simulink model "auto_pilot_udp"  (R2022b)
settings: Solver=FixedStepAuto  StartTime=0.0  StopTime=Inf  FixedStep=0.001  RelTol=1e-3  EnableMultiTasking=on
InitFcn:
  | clear mex
model workspace (MAT data in the model file):
  worldsim_instance : object (value not decoded)
values from neighbouring files (symbols this model uses):
  ACC_Adaptive_D = 0    [AutoPilot_parameters.m]    (also in ap_ini_param.mat; ap_initialModel.sldd = 0.0)
  ACC_Adaptive_I = 0    [AutoPilot_parameters.m]    (also in ap_ini_param.mat; ap_initialModel.sldd = 0.0)
  ACC_Adaptive_P = [5 7.5]    [AutoPilot_parameters.m]    (also in ap_ini_param.mat; ap_initialModel.sldd = 5.0 7.5)
  ACC_Classic_I = 5    [AutoPilot_parameters.m]    (also in ap_ini_param.mat; ap_initialModel.sldd = 5.0)
  ACC_Classic_P = 15    [AutoPilot_parameters.m]    (also in ap_ini_param.mat; ap_initialModel.sldd = 15.0)
  ACC_MaxBrake = 50    [AutoPilot_parameters.m]    (also in ap_ini_param.mat; ap_initialModel.sldd = 50.0)
  ACC_MaxThrottle = 130    [AutoPilot_parameters.m]    (also in ap_ini_param.mat = 80; ap_initialModel.sldd = 130.0)
  ACC_Module_Activity_Flag = 1    [AutoPilot_parameters.m]    (also in ap_ini_param.mat; ap_initialModel.sldd = 1.0)
  ACC_Ready_Speed = 30    [AutoPilot_parameters.m]    (also in ap_ini_param.mat; ap_initialModel.sldd = 30.0)
  ACC_SensorMaxDistance = 250    [AutoPilot_parameters.m]    (also in ap_ini_param.mat = 120; ap_initialModel.sldd = 250.0)
  ACC_Speed_Distance_control = 3    [AutoPilot_parameters.m]    (also in ap_ini_param.mat; ap_initialModel.sldd = 3.0)
  ACC_Speed_Distance_Gain = [0.1 0.15 0.2 0.25]    [AutoPilot_parameters.m]    (also in ap_ini_param.mat; ap_initialModel.sldd = 0.1 0.15 0.2 0.25)
  ADAS_Control_Mode = 1    [AutoPilot_parameters.m]    (also in ap_ini_param.mat; ap_initialModel.sldd = 1.0)
  AEB_Alarm_Freq = 5    [AutoPilot_parameters.m]    (also in ap_ini_param.mat; ap_initialModel.sldd = 5.0)
  AEB_Distance_To_Collision_Brake = 5    [AutoPilot_parameters.m]    (also in ap_ini_param.mat; ap_initialModel.sldd = 5.0)
  AEB_Freq_Hz = Sensor_Freq_worldsim/2    (= 25)    [AutoPilot_parameters.m]    (also in ap_ini_param.mat; ap_initialModel.sldd = 25.0)
  AEB_Gain = [1 1]    [AutoPilot_parameters.m]    (also in ap_ini_param.mat; ap_initialModel.sldd = 1.0 1.0)
  AEB_Gain_set = 60    [AutoPilot_parameters.m]    (also in ap_ini_param.mat; ap_initialModel.sldd = 60.0)
  AEB_Gain_set_mult = 0.03    [AutoPilot_parameters.m]    (also in ap_ini_param.mat; ap_initialModel.sldd)
  AEB_Max_Decel = [8 15]    [AutoPilot_parameters.m]    (also in ap_ini_param.mat; ap_initialModel.sldd = 8.0 15.0)
  AEB_Max_Speed = 150    [AutoPilot_parameters.m]    (also in ap_ini_param.mat = 100; ap_initialModel.sldd = 150.0)
  AEB_Min_Distance_at_Stop = 1    [AutoPilot_parameters.m]    (also in ap_ini_param.mat; ap_initialModel.sldd = 1.0)
  AEB_Module_Activity_Flag = 1    [AutoPilot_parameters.m]    (also in ap_ini_param.mat; ap_initialModel.sldd = 1.0)
  AEB_Pedestrian_type = 68    [AutoPilot_parameters.m]    (also in ap_ini_param.mat; ap_initialModel.sldd = 68.0)
  AEB_Steer_Max = 180    [AutoPilot_parameters.m]    (also in ap_ini_param.mat; ap_initialModel.sldd = 180.0)
  AP_Activity_Flag = 1    [AutoPilot_parameters.m]    (also in ap_ini_param.mat; ap_initialModel.sldd = 1.0)
  AP_D = [0.3 0.3]    [AutoPilot_parameters.m]    (also in ap_ini_param.mat; ap_initialModel.sldd = 0.3 0.3)
  AP_Dyn_Rate_Limiter_Gain = 0.1    [AutoPilot_parameters.m]    (also in ap_ini_param.mat; ap_initialModel.sldd)
  AP_Dyn_Rate_Limiter_Power = 10    [AutoPilot_parameters.m]    (also in ap_ini_param.mat; ap_initialModel.sldd = 10.0)
  AP_Error_Max = 3    [AutoPilot_parameters.m]    (also in ap_ini_param.mat; ap_initialModel.sldd = 3.0)
  AP_Freq_Hz = Sensor_Freq_worldsim    (= 50)    [AutoPilot_parameters.m]    (also in ap_ini_param.mat; ap_initialModel.sldd = 50.0)
  AP_I = [0.05 0.05]    [AutoPilot_parameters.m]    (also in ap_ini_param.mat; ap_initialModel.sldd = 0.05 0.05)
  AP_Max_Error_dydt_Disable = 0.5    [AutoPilot_parameters.m]    (also in ap_ini_param.mat; ap_initialModel.sldd)
  AP_On_Request_Time = 0.01    [AutoPilot_parameters.m]    (also in ap_ini_param.mat; ap_initialModel.sldd)
  AP_P = [0.2 0.2]    [AutoPilot_parameters.m]    (also in ap_ini_param.mat; ap_initialModel.sldd = 0.2 0.2)
  AP_Steer_Error_Max = 0.7    [AutoPilot_parameters.m]    (also in ap_ini_param.mat; ap_initialModel.sldd)
  AP_Steer_Rate_Max_radps = 1    [AutoPilot_parameters.m]    (also in ap_ini_param.mat; ap_initialModel.sldd = 1.0)
  AP_Transition_Rate = 0.5    [AutoPilot_parameters.m]    (also in ap_ini_param.mat; ap_initialModel.sldd)
  butter_a = [1 -1.9911142922 0.991153595869]    [ap_ini_param.mat]    (also in ap_initialModel.sldd = 1.0 -1.9911142922016536 0.99115359586893548)
  butter_a_lka_out = 1.0 -1.5610180758007179 0.641351538057563    [ap_initialModel.sldd]
  butter_b = [9.82591682048e-06 1.9651833641e-05 9.82591682048e-06]    [ap_ini_param.mat]    (also in ap_initialModel.sldd = 9.825916820482009E-6 1.9651833640964018E-5 9.825916820482009)
  butter_b_lka_out = 0.020083365564211246 0.040166731128422492 0.020083365564211246    [ap_initialModel.sldd]
  Lane_Width = 3.7    [AutoPilot_parameters.m]    (also in ap_ini_param.mat; ap_initialModel.sldd)
  LDW_Activity_Flag = 1    [ap_ini_param.mat]    (also in ap_initialModel.sldd = 1.0)
  LDW_Freq_Hz = 50    [ap_ini_param.mat]    (also in ap_initialModel.sldd = 50.0)
  LDW_LaneGap_dydt_Warning = 50    [ap_ini_param.mat]    (also in ap_initialModel.sldd = 50.0)
  LDW_LaneGap_Warning = [0.5 0.25]    [ap_ini_param.mat]    (also in ap_initialModel.sldd = 0.5 0.25)
  LDW_Min_Speed = 60    [ap_ini_param.mat]    (also in ap_initialModel.sldd = 60.0)
  LDW_Steer_Vibration_Amplitude = 5    [ap_ini_param.mat]    (also in ap_initialModel.sldd = 5.0)
  LDW_Steer_Vibration_Freq = 25    [ap_ini_param.mat]    (also in ap_initialModel.sldd = 25.0)
  LKA_Activity_Flag = 1    [ap_ini_param.mat]    (also in ap_initialModel.sldd = 1.0)
  LKA_D = [0.2 0.3]    [ap_ini_param.mat]    (also in ap_initialModel.sldd = 0.2 0.3)
  LKA_Dyn_Rate_Limiter_Gain = 0.1    [ap_ini_param.mat]    (also in ap_initialModel.sldd)
  LKA_Dyn_Rate_Limiter_Power = 10    [ap_ini_param.mat]    (also in ap_initialModel.sldd = 10.0)
  LKA_Error_dydt_Off = 1    [ap_ini_param.mat]    (also in ap_initialModel.sldd = 1.0)
  LKA_Error_Max = 3    [ap_ini_param.mat]    (also in ap_initialModel.sldd = 3.0)
  LKA_Error_Off = 0.5    [ap_ini_param.mat]    (also in ap_initialModel.sldd)
  LKA_Freq_Hz = 50    [ap_ini_param.mat]    (also in ap_initialModel.sldd = 50.0)
  LKA_I = [0.025 0.05]    [ap_ini_param.mat]    (also in ap_initialModel.sldd = 0.025 0.05)
  LKA_Lane_Gap_Activate = [0.25 0.125]    [ap_ini_param.mat]    (also in ap_initialModel.sldd = 0.25 0.125)
  LKA_Lane_Gap_dydt_Activate = 50    [ap_ini_param.mat]    (also in ap_initialModel.sldd = 50.0)
  LKA_Min_Speed = 60    [ap_ini_param.mat]    (also in ap_initialModel.sldd = 60.0)
  LKA_On_Display_Freq = 5    [ap_ini_param.mat]    (also in ap_initialModel.sldd = 5.0)
  LKA_P = [0.1 0.2]    [ap_ini_param.mat]    (also in ap_initialModel.sldd = 0.1 0.2)
  LKA_Steer_Rate_Max_radps = 1    [ap_ini_param.mat]    (also in ap_initialModel.sldd = 1.0)
  No_Target_Display_Value = 0    [AutoPilot_parameters.m]    (also in ap_ini_param.mat; ap_initialModel.sldd = 0.0)
  radar_source = 2    [AutoPilot_parameters.m]    (also in ap_ini_param.mat; ap_initialModel.sldd = 2.0)
  Sensor_Freq_worldsim = 50    [AutoPilot_parameters.m]    (also in ap_ini_param.mat; ap_initialModel.sldd = 50.0; launcher.m)
  stop_number_collisions = 10.0    [ap_initialModel.sldd]    (also in launcher.m = 10)
  stop_speed = 0.001    [ap_initialModel.sldd]    (also in launcher.m)
  stop_time = 12.0    [ap_initialModel.sldd]    (also in launcher.m = 12)
  vehicle_width = 2.2    [AutoPilot_parameters.m]    (also in ap_ini_param.mat = 1.86; ap_initialModel.sldd)
undefined symbols (not defined in the file or in its folder): blockPlatform, HOST, light_brake_center, light_brake_left, light_brake_right
libraries: simulink x103, simwbSfunlib x35, slpidlib x5, viworldsim_lib x5
(part 4 of 5)

== system auto_pilot_udp/AP/AP_Logic/Discrete PID Controller2 ==
  In1 : Inport
  In2 : Inport  Port=2
  In4 : Inport  Port=3
  ADAS_Control_Mode : Constant  Value=ADAS_Control_Mode
  AP_D(1)(1) : Constant  Value=AP_D(1)
  AP_D(2)(1)1 : Constant  Value=AP_D(2)
  AP_I(1)(1) : Constant  Value=AP_I(1)
  AP_I(2)(1)1 : Constant  Value=AP_I(2)
  AP_P(1)(1) : Constant  Value=AP_P(1)
  AP_P(2)(1)1 : Constant  Value=AP_P(2)
  Constant : Constant  Value=0
  Demux : Demux  Outputs=3
  Discrete PID Controller2 : slpidlib/PID Controller  Controller=PID  Form=Parallel  TimeDomain=Discrete-time  UseExternalTs=off  SampleTime=1/AP_Freq_Hz  IntegratorMethod=Forward Euler  FilterMethod=Forward Euler  ControllerParametersSource=external  P=AP_P  I=AP_I  UseKiTs=off  D=AP_D  N=100  UseFilter=off  TunerSelectOption=Transfer Function Based (PID Tuner App)  InitialConditionSource=external  InitialConditionForIntegrator=0  InitialConditionForFilter=0  DifferentiatorICPrevScaledInput=0  ExternalReset=either  TrackingMode=off  Kt=1  LimitOutput=off  SatLimitsSource=internal  UpperSaturationLimit=ACC_MaxThrottle  LowerSaturationLimit=-ACC_MaxBrake  LinearizeAsGain=off  AntiWindupMode=back-calculation  Kb=1  LimitIntegrator=off  UpperIntegratorSaturationLimit=inf  LowerIntegratorSaturationLimit=-inf  POutMin=[]  POutMax=[]  IOutMin=[]  IOutMax=[]  DOutMin=[]  DOutMax=[]  NOutMin=[]  NOutMax=[]  SumOutMin=[]  SumOutMax=[]  SaturationOutMin=[]  SaturationOutMax=[]  PParamMin=[]  PParamMax=[]  IParamMin=[]  IParamMax=[]  DParamMin=[]  DParamMax=[]  NParamMin=[]  NParamMax=[]  KbParamMin=[]  KbParamMax=[]  KtParamMin=[]  KtParamMax=[]  KbOutMin=[]  KbOutMax=[]  KtOutMin=[]  KtOutMax=[]  IntegratorOutMin=[]  IntegratorOutMax=[]  FilterOutMin=[]  FilterOutMax=[]  SumI1OutMin=[]  SumI1OutMax=[]  SumI2OutMin=[]  SumI2OutMax=[]  SumI3OutMin=[]  SumI3OutMax=[]  SumI4OutMin=[]  SumI4OutMax=[]  SumDOutMin=[]  SumDOutMax=[]  DifferentiatorOutMin=[]  DifferentiatorOutMax=[]  FilterDiffOutCoefMin=[]  FilterDiffOutCoefMax=[]  ReciprocalOutMin=[]  ReciprocalOutMax=[]  SumDenOutMin=[]  SumDenOutMax=[]  SumNumOutMin=[]  SumNumOutMax=[]  DivideOutMin=[]  DivideOutMax=[]  UdiffTsProdOutMin=[]  UdiffTsProdOutMax=[]  NTsProdOutMin=[]  NTsProdOutMax=[]  UintegralTsProdOutMin=[]  UintegralTsProdOutMax=[]  UngainTsProdOutMin=[]  UngainTsProdOutMax=[]  ClampingZeroOutDataTypeStr=Inherit: Inherit via back propagation  ClampingZeroOutMin=[]  ClampingZeroOutMax=[]  FilterDenConstantOutDataTypeStr=Inherit: Inherit via back propagation  FilterDenConstantOutMin=[]  FilterDenConstantOutMax=[]  PCopyOutDataTypeStr=Inherit: Inherit via back propagation  PCopyOutMin=[]  PCopyOutMax=[]  NCopyOutDataTypeStr=Inherit: Inherit via back propagation  NCopyOutMin=[]  NCopyOutMax=[]  IntegratorContinuousStateAttributes=''  IntegratorStateMustResolveToSignalObject=off  IntegratorRTWStateStorageClass=Auto  FilterContinuousStateAttributes=''  FilterStateMustResolveToSignalObject=off  FilterRTWStateStorageClass=Auto  ParallelPVariant=ExternalParameters  IdealPVariant=Disabled  IVariant=ExternalParameters  DVariant=ExternalParameters  IntegratorVariant=Discrete  SatVariant=Disabled  AWVariant=Passthrough  PCopyVariant=Disabled  TRVariant=Disabled  FdbkBlocksVariant=Forward  IdealPFdbkVariant=Disabled  SatFdbkVariant=Disabled  DerivativeFilterVariant=Differentiator  NVariant=Passthrough  NCopyVariant=Disabled_SignalSpec  FilterICVariant=ExternalICs  IntegratorICVariant=ExternalICs  ExternalResetVariant=ExternalReset  TRSumVariant=Passthrough  SumFdbkVariant=Disabled  SumVariant=Sum_PID  TsampFilterVariant=InternalTs  TsampNgainVariant=Passthrough  TsampIntegralVariant=Passthrough  ExternalSaturationOutDataTypeStr=Inherit: Same as second input
  Multiport Switch : MultiPortSwitch  Inputs=2  DataPortForDefault=Additional data port  DiagnosticForDefault=None  SaturateOnIntegerOverflow=off  InputSameDT=off
  Mux : Mux  Inputs=3
  Mux1 : Mux  Inputs=3
  Out1 : Outport  VectorParamsAs1DForOutWhenUnconnected=off
  wires:
  Constant/1 -> Discrete PID Controller2/7
  In2/1 -> Discrete PID Controller2/5
  Discrete PID Controller2/1 -> Out1/1
  In4/1 -> Discrete PID Controller2/6
  In1/1 -> Discrete PID Controller2/1
  AP_P(1)(1)/1 -> Mux/1
  ADAS_Control_Mode/1 -> Multiport Switch/1
  Mux1/1 -> Multiport Switch/3
  Mux/1 -> Multiport Switch/4, Multiport Switch/2
  AP_I(1)(1)/1 -> Mux/2
  AP_D(1)(1)/1 -> Mux/3
  AP_P(2)(1)1/1 -> Mux1/1
  AP_I(2)(1)1/1 -> Mux1/2
  AP_D(2)(1)1/1 -> Mux1/3
  Multiport Switch/1 -> Demux/1
  Demux/2 -> Discrete PID Controller2/3
  Demux/1 -> Discrete PID Controller2/2
  Demux/3 -> Discrete PID Controller2/4

== system auto_pilot_udp/AP/AP_Logic/Subsystem ==
  Clock : Inport
  Input_Signal : Inport  Port=2
  Delay : Delay  DelayLength=1000/AP_Freq_Hz  InitialCondition=-1/AP_Freq_Hz
  Delay1 : Delay  DelayLength=1000/AP_Freq_Hz
  Delay2 : Delay  DelayLength=1000/AP_Freq_Hz
  Lookup Table Dynamic : simulink/Lookup Tables/Lookup Table Dynamic  LookUpMeth=Interpolation-Use End Values  OutDataType=fixdt('double')  OutScaling=[]  OutputDataTypeScalingMode=Specify via dialog  OutDataTypeStr=fixdt('double')  DoSatur=off
  Vector Concatenate : Concatenate
  Vector Concatenate1 : Concatenate
  Zero-Order Hold1 : ZeroOrderHold  SampleTime=1/AP_Freq_Hz
  Zero-Order Hold2 : ZeroOrderHold  SampleTime=1/AP_Freq_Hz
  Zero-Order Hold3 : ZeroOrderHold  SampleTime=1e-3
  Zero-Order Hold4 : ZeroOrderHold  SampleTime=1e-3
  1kHz_Interpolation : Outport  VectorParamsAs1DForOutWhenUnconnected=off
  wires:
  Input_Signal/1 -> Zero-Order Hold1/1
  Zero-Order Hold1/1 -> Zero-Order Hold4/1
  Zero-Order Hold3/1 -> Delay/1, Vector Concatenate/2
  Zero-Order Hold2/1 -> Zero-Order Hold3/1
  Delay/1 -> Vector Concatenate/1
  Delay1/1 -> Lookup Table Dynamic/1
  Delay2/1 -> Vector Concatenate1/1
  Zero-Order Hold4/1 -> Delay2/1, Vector Concatenate1/2
  Vector Concatenate1/1 -> Lookup Table Dynamic/3
  Vector Concatenate/1 -> Lookup Table Dynamic/2
  Clock/1 -> Delay1/1, Zero-Order Hold2/1
  Lookup Table Dynamic/1 -> 1kHz_Interpolation/1

== system auto_pilot_udp/INPUT/Inputs for CRT/Clutch_manager ==
  throttle : Inport
  Cast To Double : DataTypeConversion  OutDataTypeStr=double  SaturateOnIntegerOverflow=off  RndMeth=Floor
  Compare To Constant4 : simulink/Logic and Bit Operations/Compare To Constant  relop===  const=0  OutDataTypeStr=boolean
  clutch : Outport
  wires:
  Compare To Constant4/1 -> Cast To Double/1
  Cast To Double/1 -> clutch/1  "clutch"
  throttle/1 -> Compare To Constant4/1

== system auto_pilot_udp/OUTPUT/WorldSim_Sensor_Outputs/Radar_selection ==
  note: assignement
  Bus Creator : BusCreator  Inputs=12
  Constant1 : Constant  Value=radar_source
  Demux : Demux  Outputs=3
  Demux1 : Demux
  Demux2 : Demux
  Demux3 : Demux
  Multiport Switch : MultiPortSwitch  Inputs=2  SaturateOnIntegerOverflow=off  InputSameDT=off
  Terminator : Terminator
  tag scope: SensorTargets_300000_azimuthInSensor_mux=global, SensorTargets_300000_distanceToCollision_mux=global, SensorTargets_300000_id_mux=global, SensorTargets_300000_type_mux=global, SensorTargets_300001_azimuthInSensor_mux=global, SensorTargets_300001_distanceToCollision_mux=global, SensorTargets_300001_id_mux=global, SensorTargets_300001_type_mux=global, SensorTargets_300002_azimuthInSensor_mux=global, SensorTargets_300002_distanceToCollision_mux=global, SensorTargets_300002_id_mux=global, SensorTargets_300002_type_mux=global
  wires:
  [radar_virtual] -> Multiport Switch/3
  [radar_multiagent] -> Multiport Switch/2
  Constant1/1 -> Multiport Switch/1
  Multiport Switch/1 -> Demux/1
  Demux1/1 -> [SensorTargets_300000_id_mux]
  Demux3/4 -> [SensorTargets_300002_type_mux]
  Demux3/1 -> [SensorTargets_300002_id_mux]
  Demux1/4 -> [SensorTargets_300000_type_mux]
  Demux3/2 -> [SensorTargets_300002_distanceToCollision_mux]
  Demux2/3 -> [SensorTargets_300001_azimuthInSensor_mux]
  Demux1/2 -> [SensorTargets_300000_distanceToCollision_mux]
  Demux/1 -> Demux1/1
  Demux1/3 -> [SensorTargets_300000_azimuthInSensor_mux]
  Demux2/2 -> [SensorTargets_300001_distanceToCollision_mux]
  Demux3/3 -> [SensorTargets_300002_azimuthInSensor_mux]
  Demux2/4 -> [SensorTargets_300001_type_mux]
  Demux/3 -> Demux3/1
  Demux/2 -> Demux2/1
  Demux2/1 -> [SensorTargets_300001_id_mux]
  [SensorTargets_300000_id_mux] -> Bus Creator/1
  [SensorTargets_300000_distanceToCollision_mux] -> Bus Creator/2
  [SensorTargets_300000_azimuthInSensor_mux] -> Bus Creator/3
  [SensorTargets_300000_type_mux] -> Bus Creator/4
  [SensorTargets_300001_id_mux] -> Bus Creator/5
  [SensorTargets_300001_distanceToCollision_mux] -> Bus Creator/6
  [SensorTargets_300001_azimuthInSensor_mux] -> Bus Creator/7
  [SensorTargets_300001_type_mux] -> Bus Creator/8
  [SensorTargets_300002_id_mux] -> Bus Creator/9
  [SensorTargets_300002_distanceToCollision_mux] -> Bus Creator/10
  [SensorTargets_300002_azimuthInSensor_mux] -> Bus Creator/11
  [SensorTargets_300002_type_mux] -> Bus Creator/12
  Bus Creator/1 -> Terminator/1

== system auto_pilot_udp/OUTPUT/WorldSim_Sensor_Outputs/Subsystem ==
  Multiagent_radar_matrix [dimension: 64x7] : Inport
  Virtual_camera_radar_matrix [dimension: 10x10] : Inport  Port=2
  BSD_virtual_camera_matrix [dimension: 10x10] : Inport  Port=3
  Left_lane_distance [dimension: 1x1] : Inport  Port=4
  Right_lane_distance [dimension: 1x1] : Inport  Port=5
  Lane_detector_message_count [dimension: 1x1] : Inport  Port=6
  Semitrack : Constant  Value=vehicle_width/2
  Terminator : Terminator
  Terminator1 : Terminator
  bsd setection from ostacle recognition : Subsystem
  lane marking acquisition : Subsystem
  "multiagent radar SimpleRadar_... are single double representing id, yaw, range, power_db, range_rate, yaw_rate, status" : Subsystem
  "obstacle detection " : Subsystem
  tag scope: frame_worldsim_left=global, frame_worldsim_right=global
  wires:
  Semitrack/1 -> lane marking acquisition/1(Semitrack), bsd setection from ostacle recognition/1(semitrack)
  Virtual_camera_radar_matrix [dimension: 10x10]/1 -> "obstacle detection "/1(Virtual_camera_obstacle_matrix)
  BSD_virtual_camera_matrix [dimension: 10x10]/1 -> bsd setection from ostacle recognition/2(BSD_matrix_obstalces)
  Left_lane_distance [dimension: 1x1]/1 -> lane marking acquisition/2(Left_lane_marking)
  Right_lane_distance [dimension: 1x1]/1 -> lane marking acquisition/3(Right_lane_marking)
  Multiagent_radar_matrix [dimension: 64x7]/1 -> "multiagent radar SimpleRadar_... are single double representing id, yaw, range, power_db, range_rate, yaw_rate, status"/1(Virtual_radar_obstacle_matrix)
  Lane_detector_message_count [dimension: 1x1]/1 -> [frame_worldsim_right], [frame_worldsim_left]
  [frame_worldsim_left] -> Terminator/1
  [frame_worldsim_right] -> Terminator1/1

== system auto_pilot_udp/VI-WorldSim Lights Manager/Lights/Default Lights Bus ==
  Bus Creator : BusCreator  Inputs=15
  Constant{,1..12,14..15} (15 alike) : Constant  Value=0
  Out1 : Outport  VectorParamsAs1DForOutWhenUnconnected=off
  wires:
  Bus Creator/1 -> Out1/1
  Constant12/1 -> Bus Creator/15  "light_daytime"
  Constant14/1 -> Bus Creator/13  "light_brake_center"
  Constant8/1 -> Bus Creator/9  "light_tail_left"
  Constant15/1 -> Bus Creator/14  "light_reverse"
  Constant2/1 -> Bus Creator/3  "light_high_beam_left"
  Constant5/1 -> Bus Creator/6  "light_indicator_right"
  Constant3/1 -> Bus Creator/4  "light_high_beam_right"
  Constant7/1 -> Bus Creator/8  "light_fog_right"
  Constant6/1 -> Bus Creator/7  "light_fog_left"
  Constant4/1 -> Bus Creator/5  "light_indicator_left"
  Constant1/1 -> Bus Creator/2  "light_low_beam_right"
  Constant/1 -> Bus Creator/1  "light_low_beam_left"
  Constant9/1 -> Bus Creator/10  "light_tail_right"
  Constant11/1 -> Bus Creator/12  "light_brake_right"
  Constant10/1 -> Bus Creator/11  "light_brake_left"

== system auto_pilot_udp/ACC/ACC_Logic/ACC_Speed_Controller/ACC_Speed_Distance_Gain ==
  note: this should be used when no varying distance is used
  In1 : Inport
  ACC_Speed_Distance_Gain : Gain  Gain=ACC_Speed_Distance_Gain(1)
  ACC_Speed_Distance_Gain1 : Gain  Gain=ACC_Speed_Distance_Gain(2)
  ACC_Speed_Distance_Gain2 : Gain  Gain=ACC_Speed_Distance_Gain(3)
  ACC_Speed_Distance_Gain3 : Gain  Gain=ACC_Speed_Distance_Gain(4)
  ADAS_Control_Mode : Constant  Value=ADAS_Control_Mode
  Cast To Double : DataTypeConversion  OutDataTypeStr=double  SaturateOnIntegerOverflow=off  RndMeth=Floor
  Detect Increase : simulink/Logic and Bit Operations/Detect Increase  vinit=0.0  OutDataTypeStr=boolean
  Detect Increase1 : simulink/Logic and Bit Operations/Detect Increase  vinit=0.0  OutDataTypeStr=boolean
  Gain : Gain  Gain=-1
  Memory : Memory  InitialCondition=ACC_Speed_Distance_control
  Multiport Switch : MultiPortSwitch  Inputs=4  DataPortForDefault=Additional data port  DiagnosticForDefault=None  SaturateOnIntegerOverflow=off  InputSameDT=off
  Saturation : Saturate  UpperLimit=4  LowerLimit=1
  Sum : Sum  Inputs=+++
  Terminator : Terminator
  Terminator1 : Terminator
  Out1 : Outport  VectorParamsAs1DForOutWhenUnconnected=off
  tag scope: ACC_distance_step=global
  wires:
  Multiport Switch/1 -> Out1/1
  In1/1 -> ACC_Speed_Distance_Gain3/1, ACC_Speed_Distance_Gain2/1, ACC_Speed_Distance_Gain1/1, ACC_Speed_Distance_Gain/1
  ACC_Speed_Distance_Gain/1 -> Multiport Switch/2
  ACC_Speed_Distance_Gain1/1 -> Multiport Switch/6, Multiport Switch/3
  ACC_Speed_Distance_Gain2/1 -> Multiport Switch/4
  ACC_Speed_Distance_Gain3/1 -> Multiport Switch/5
  [mode_minus] -> Detect Increase/1
  Detect Increase/1 -> Gain/1
  [mode_plus] -> Detect Increase1/1
  Sum/1 -> Multiport Switch/1, Memory/1, Cast To Double/1
  Memory/1 -> Saturation/1
  Saturation/1 -> Sum/3
  Detect Increase1/1 -> Sum/2
  Gain/1 -> Sum/1
  ADAS_Control_Mode/1 -> Terminator/1
  Cast To Double/1 -> [ACC_distance_step]
  [ACC_distance_step] -> Terminator1/1

== system auto_pilot_udp/ACC/ACC_Logic/ACC_Speed_Controller/tACC_PID ==
  In1 : Inport
  In2 : Inport  Port=2
  ACC_Adaptive_P : Constant  Value=ACC_Adaptive_P(1)
  ACC_Adaptive_P2 : Constant  Value=ACC_Adaptive_P(2)
  ADAS_Control_Mode : Constant  Value=ADAS_Control_Mode
  Constant : Constant  Value=0
  Multiport Switch : MultiPortSwitch  Inputs=2  DataPortForDefault=Additional data port  DiagnosticForDefault=None  SaturateOnIntegerOverflow=off  InputSameDT=off
  tACC_PID : slpidlib/PID Controller  Controller=PID  Form=Parallel  TimeDomain=Discrete-time  UseExternalTs=off  SampleTime=-1  IntegratorMethod=Forward Euler  FilterMethod=Forward Euler  ControllerParametersSource=external  P=ACC_Adaptive_P  I=ACC_Adaptive_I  UseKiTs=off  D=ACC_Adaptive_D  N=100  UseFilter=off  TunerSelectOption=Transfer Function Based (PID Tuner App)  InitialConditionSource=internal  InitialConditionForIntegrator=0  InitialConditionForFilter=0  DifferentiatorICPrevScaledInput=0  ExternalReset=either  TrackingMode=off  Kt=1  LimitOutput=on  SatLimitsSource=internal  UpperSaturationLimit=ACC_MaxThrottle  LowerSaturationLimit=-ACC_MaxBrake  LinearizeAsGain=off  AntiWindupMode=back-calculation  Kb=1  LimitIntegrator=off  UpperIntegratorSaturationLimit=inf  LowerIntegratorSaturationLimit=-inf  POutMin=[]  POutMax=[]  IOutMin=[]  IOutMax=[]  DOutMin=[]  DOutMax=[]  NOutMin=[]  NOutMax=[]  SumOutMin=[]  SumOutMax=[]  SaturationOutMin=[]  SaturationOutMax=[]  PParamMin=[]  PParamMax=[]  IParamMin=[]  IParamMax=[]  DParamMin=[]  DParamMax=[]  NParamMin=[]  NParamMax=[]  KbParamMin=[]  KbParamMax=[]  KtParamMin=[]  KtParamMax=[]  KbOutMin=[]  KbOutMax=[]  KtOutMin=[]  KtOutMax=[]  IntegratorOutMin=[]  IntegratorOutMax=[]  FilterOutMin=[]  FilterOutMax=[]  SumI1OutMin=[]  SumI1OutMax=[]  SumI2OutMin=[]  SumI2OutMax=[]  SumI3OutMin=[]  SumI3OutMax=[]  SumI4OutMin=[]  SumI4OutMax=[]  SumDOutMin=[]  SumDOutMax=[]  DifferentiatorOutMin=[]  DifferentiatorOutMax=[]  FilterDiffOutCoefMin=[]  FilterDiffOutCoefMax=[]  ReciprocalOutMin=[]  ReciprocalOutMax=[]  SumDenOutMin=[]  SumDenOutMax=[]  SumNumOutMin=[]  SumNumOutMax=[]  DivideOutMin=[]  DivideOutMax=[]  UdiffTsProdOutMin=[]  UdiffTsProdOutMax=[]  NTsProdOutMin=[]  NTsProdOutMax=[]  UintegralTsProdOutMin=[]  UintegralTsProdOutMax=[]  UngainTsProdOutMin=[]  UngainTsProdOutMax=[]  ClampingZeroOutDataTypeStr=Inherit: Inherit via back propagation  ClampingZeroOutMin=[]  ClampingZeroOutMax=[]  FilterDenConstantOutDataTypeStr=Inherit: Inherit via back propagation  FilterDenConstantOutMin=[]  FilterDenConstantOutMax=[]  PCopyOutDataTypeStr=Inherit: Inherit via back propagation  PCopyOutMin=[]  PCopyOutMax=[]  NCopyOutDataTypeStr=Inherit: Inherit via back propagation  NCopyOutMin=[]  NCopyOutMax=[]  IntegratorContinuousStateAttributes=''  IntegratorStateMustResolveToSignalObject=off  IntegratorRTWStateStorageClass=Auto  FilterContinuousStateAttributes=''  FilterStateMustResolveToSignalObject=off  FilterRTWStateStorageClass=Auto  ParallelPVariant=ExternalParameters  IdealPVariant=Disabled  IVariant=ExternalParameters  DVariant=ExternalParameters  IntegratorVariant=Discrete  SatVariant=Enabled  AWVariant=BackCalculation  PCopyVariant=Disabled  TRVariant=Disabled  FdbkBlocksVariant=Forward  IdealPFdbkVariant=Disabled  SatFdbkVariant=Disabled  DerivativeFilterVariant=Differentiator  NVariant=Passthrough  NCopyVariant=Disabled_SignalSpec  FilterICVariant=InternalICsDifferentiator  IntegratorICVariant=InternalICs  ExternalResetVariant=ExternalReset  TRSumVariant=Passthrough  SumFdbkVariant=Disabled  SumVariant=Sum_PID  TsampFilterVariant=InternalTs  TsampNgainVariant=Passthrough  TsampIntegralVariant=Passthrough  ExternalSaturationOutDataTypeStr=Inherit: Same as second input
  Out1 : Outport  VectorParamsAs1DForOutWhenUnconnected=off
  wires:
  tACC_PID/1 -> Out1/1
  In1/1 -> tACC_PID/1
  In2/1 -> tACC_PID/5
  ACC_Adaptive_P/1 -> Multiport Switch/4, Multiport Switch/2
  ADAS_Control_Mode/1 -> Multiport Switch/1
  ACC_Adaptive_P2/1 -> Multiport Switch/3
  Multiport Switch/1 -> tACC_PID/2
  Constant/1 -> tACC_PID/3, tACC_PID/4

== system auto_pilot_udp/ACC/ACC_Logic/ACC_Target_Acquisition/SensorTargets_300000_ClosestTargetDistance ==
  ACC_SensorMaxDistance : Constant  Value=ACC_SensorMaxDistance + 1
  Abs : Abs  SaturateOnIntegerOverflow=off
  MinMax : MinMax
  Switch : Switch  Criteria=u2 > Threshold  SaturateOnIntegerOverflow=off  InputSameDT=off
  Switch1 : Switch  Criteria=u2 > Threshold  Threshold=0.02  SaturateOnIntegerOverflow=off  InputSameDT=off
  tag scope: SensorTargets_300000_ClosestTargetDistance=global
  wires:
  [SensorTargets_300000_distanceToCollision_mux] -> Switch/1
  ACC_SensorMaxDistance/1 -> Switch/3
  MinMax/1 -> [SensorTargets_300000_ClosestTargetDistance]
  Switch1/1 -> Switch/2
  [SensorTargets_300000_InStraightLane_mux] -> Switch1/3
  [SensorTargets_300000_InCurvedLane_mux] -> Switch1/1
  [ACC_Input_Front_Axle_Steer] -> Abs/1
  Abs/1 -> Switch1/2
  Switch/1 -> MinMax/1

== system auto_pilot_udp/ACC/ACC_Logic/ACC_Target_Acquisition/SensorTargets_300000_ClosestTargetId ==
  note: if ws_radar is used or simple multiagent radar is used
  AND : Logic  AllPortsSameDT=off  OutDataTypeStr=boolean
  Compare To Constant : simulink/Logic and Bit Operations/Compare To Constant  relop=~=  const=1  OutDataTypeStr=boolean
  Compare To Constant1 : simulink/Logic and Bit Operations/Compare To Constant  relop=~=  const=1  OutDataTypeStr=boolean
  Compare To Constant2 : simulink/Logic and Bit Operations/Compare To Constant  relop===  const=121  OutDataTypeStr=boolean
  Compare To Constant3 : simulink/Logic and Bit Operations/Compare To Constant  relop===  const=3  OutDataTypeStr=boolean
  Constant : Constant  Value=0
  Constant1 : Constant  Value=radar_source
  Logical Operator : Logic  Operator=OR  Inputs=4  AllPortsSameDT=off  OutDataTypeStr=boolean
  Logical Operator1 : Logic  Operator=OR  AllPortsSameDT=off  OutDataTypeStr=boolean
  MinMax : MinMax  Function=max
  No_Target_Display_Value : Constant  Value=No_Target_Display_Value
  Product : Product
  Relational Operator : RelationalOperator  Operator===  OutDataTypeStr=boolean  InputSameDT=off
  Relational Operator1 : RelationalOperator  Operator=isNaN  OutDataTypeStr=boolean  InputSameDT=off
  Relational Operator2 : RelationalOperator  Operator=isInf  OutDataTypeStr=boolean  InputSameDT=off
  Switch : Switch  Criteria=u2 > Threshold  SaturateOnIntegerOverflow=off  InputSameDT=off
  Switch1 : Switch  Criteria=u2 > Threshold  SaturateOnIntegerOverflow=off  InputSameDT=off
  tag scope: ACC_Target_id=global
  wires:
  Product/1 -> MinMax/1
  Relational Operator/1 -> Product/2
  [SensorTargets_300000_id_mux] -> Product/1
  [SensorTargets_300000_ClosestTargetDistance] -> Relational Operator/2
  [SensorTargets_300000_distanceToCollision_mux] -> Relational Operator/1
  No_Target_Display_Value/1 -> Switch/1
  MinMax/1 -> Relational Operator2/1, Relational Operator1/1, Switch/3
  Switch/1 -> [ACC_Target_id]
  Logical Operator/1 -> Switch/2
  Relational Operator1/1 -> Logical Operator/3
  Relational Operator2/1 -> Logical Operator/2
  Compare To Constant/1 -> Logical Operator/4
  [ACC_Active] -> Logical Operator1/2
  [ACC_Ready] -> Logical Operator1/1
  Logical Operator1/1 -> Compare To Constant/1
  [SimpleRadar_status] -> Compare To Constant1/1
  Compare To Constant1/1 -> Switch1/3
  [SensorTargets_300000_ClosestTargetDistance] -> Compare To Constant2/1
  Compare To Constant2/1 -> AND/1
  Constant1/1 -> Compare To Constant3/1
  Compare To Constant3/1 -> AND/2, Switch1/2
  AND/1 -> Switch1/1
  Switch1/1 -> Logical Operator/1
  Constant/1 -> [SimpleRadar_status]

== system auto_pilot_udp/ACC/ACC_Logic/ACC_Target_Acquisition/SensorTargets_300000_InCurvedLane_mux ==
  Abs : Abs  SaturateOnIntegerOverflow=off
  Constant : Constant  Value=vehicle_width*0.8
  Gain : Gain
  Gain1 : Gain  Gain=1.3
  Lane_Width/2 : Constant  Value=Lane_Width/2
  Logical Operator : Logic  AllPortsSameDT=off  OutDataTypeStr=boolean
  MATLAB Function : MATLAB Function  TreatAsAtomicUnit=on
  MinMax : MinMax  Function=max
  Relational Operator : RelationalOperator  Operator=<  OutDataTypeStr=boolean  InputSameDT=off
  Relational Operator1 : RelationalOperator  Operator=>  OutDataTypeStr=boolean  InputSameDT=off
  Sum : Sum
  Sum1 : Sum  Inputs=-+
  Terminator : Terminator
  Terminator1 : Terminator
  Wrap To Zero : simulink/Discontinuities/Wrap To Zero  Threshold=10000
  Wrap To Zero1 : simulink/Discontinuities/Wrap To Zero  Threshold=10000
  tag scope: ACC_CurveRadius=global, ACC_CurveRadius_Target=global, SensorTargets_300000_InCurvedLane_mux=global
  wires:
  MATLAB Function/1(Radius) -> Abs/1
  MATLAB Function/2(Rn) -> Wrap To Zero1/1, Relational Operator/2, Relational Operator1/2
  Lane_Width/2/1 -> Gain1/1
  Sum1/1 -> Relational Operator/1
  Sum/1 -> Relational Operator1/1
  Relational Operator1/1 -> Logical Operator/1
  Relational Operator/1 -> Logical Operator/2
  Logical Operator/1 -> [SensorTargets_300000_InCurvedLane_mux]
  [Vehicle_wheelbase] -> MATLAB Function/2(wheelbase)
  [ACC_Input_Front_Axle_Steer] -> Gain/1
  [SensorTargets_300000_LateralDistance_mux] -> MATLAB Function/4(SensorTargets_300000_LateralDistance)
  [SensorTargets_300000_LongitudinalDistance_mux] -> MATLAB Function/3(SensorTargets_300000_LongitudinalDistance)
  Gain/1 -> MATLAB Function/1(Front_Axle_Steer)
  Wrap To Zero/1 -> [ACC_CurveRadius]
  Abs/1 -> Wrap To Zero/1, Sum/1, Sum1/2
  Wrap To Zero1/1 -> MinMax/1
  MinMax/1 -> [ACC_CurveRadius_Target]
  Gain1/1 -> Sum1/1, Sum/2
  Constant/1 -> [Vehicle_wheelbase]
  [ACC_CurveRadius_Target] -> Terminator/1
  [ACC_CurveRadius] -> Terminator1/1

== system auto_pilot_udp/ACC/ACC_Logic/ACC_Target_Acquisition/SensorTargets_300000_InStraightLane_mux ==
  Abs : Abs  SaturateOnIntegerOverflow=off
  Compare_to_Lane_Width_div2 : simulink/Logic and Bit Operations/Compare To Constant  relop=<=  const=Lane_Width/2  OutDataTypeStr=boolean
  tag scope: SensorTargets_300000_InStraightLane_mux=global
  wires:
  Compare_to_Lane_Width_div2/1 -> [SensorTargets_300000_InStraightLane_mux]
  Abs/1 -> Compare_to_Lane_Width_div2/1
  [SensorTargets_300000_LateralDistance_mux] -> Abs/1

== system auto_pilot_udp/ACC/ACC_Logic/ACC_Target_Acquisition/SensorTargets_300000_LateralDistance_mux ==
  Target_Lateral_Position : MATLAB Function  TreatAsAtomicUnit=on
  tag scope: SensorTargets_300000_LateralDistance_mux=global
  wires:
  Target_Lateral_Position/1(Target_Lateral_Position) -> [SensorTargets_300000_LateralDistance_mux]
  [SensorTargets_300000_distanceToCollision_mux] -> Target_Lateral_Position/1(Target_distance)
  [SensorTargets_300000_azimuthInSensor_mux] -> Target_Lateral_Position/2(Target_azimuth)

== system auto_pilot_udp/ACC/ACC_Logic/ACC_Target_Acquisition/SensorTargets_300000_LongitudinalDistance_mux ==
  Target_Longitudinal_Position : MATLAB Function  TreatAsAtomicUnit=on
  tag scope: SensorTargets_300000_LongitudinalDistance_mux=global
  wires:
  [SensorTargets_300000_distanceToCollision_mux] -> Target_Longitudinal_Position/1(Target_distance)
  [SensorTargets_300000_azimuthInSensor_mux] -> Target_Longitudinal_Position/2(Target_azimuth)
  Target_Longitudinal_Position/1(Target_Longitudinal_Position) -> [SensorTargets_300000_LongitudinalDistance_mux]

== system auto_pilot_udp/AEB/AEB_Logic/Target_XY_TimeToCollision/Target_Collision_Identifier_mux    ==
  Target_Y_Left_TimeToCollision : Inport
  Target_Y_Right_TimeToCollision : Inport  Port=2
  Target_X_TimeToCollision : Inport  Port=3
  Constant : Constant  Value=AEB_Gain_set
  Constant1 : Constant
  Gain : Gain  Gain=AEB_Gain(1)
  Gain1 : Gain  Gain=AEB_Gain(2)
  Gain2 : Gain  Gain=AEB_Gain_set_mult
  Logical Operator : Logic  AllPortsSameDT=off  OutDataTypeStr=boolean
  MinMax : MinMax  Inputs=2
  MinMax1 : MinMax  Function=max  Inputs=2
  Product : Product
  Product1 : Product
  Rate Transition : RateTransition  OutPortSampleTime=1/AEB_Freq_Hz
  Rate Transition1 : RateTransition  OutPortSampleTime=1/AEB_Freq_Hz
  Relational Operator : RelationalOperator  Operator=>  OutDataTypeStr=boolean  InputSameDT=off
  Relational Operator1 : RelationalOperator  Operator=<  OutDataTypeStr=boolean  InputSameDT=off
  Saturation : Saturate  UpperLimit=1.7  LowerLimit=0.8
  Sum : Sum  Inputs=+-
  Sum1 : Sum
  Target_Collision_Identifier : Outport  VectorParamsAs1DForOutWhenUnconnected=off
  wires:
  Relational Operator1/1 -> Logical Operator/1
  Relational Operator/1 -> Logical Operator/2
  MinMax/1 -> Gain/1
  Target_Y_Right_TimeToCollision/1 -> MinMax/2, MinMax1/2
  Target_X_TimeToCollision/1 -> Relational Operator1/2, Relational Operator/2
  Target_Y_Left_TimeToCollision/1 -> MinMax/1, MinMax1/1
  MinMax1/1 -> Gain1/1
  Constant/1 -> Sum/1
  [Vehicle_Speed] -> Rate Transition/1
  Gain/1 -> Product/2
  Gain1/1 -> Product1/2
  Constant1/1 -> Sum1/1
  Sum/1 -> Gain2/1
  Gain2/1 -> Sum1/2
  Sum1/1 -> Saturation/1
  Rate Transition/1 -> Sum/2
  Logical Operator/1 -> Rate Transition1/1
  Rate Transition1/1 -> Target_Collision_Identifier/1
  Product/1 -> Relational Operator1/1
  Saturation/1 -> Product1/1, Product/1
  Product1/1 -> Relational Operator/1

== system auto_pilot_udp/AEB/AEB_Logic/Target_XY_TimeToCollision/Target_X_TimeToCollision_mux ==
  Target_X_Distance : Inport
  Discrete Derivative : simulink/Discrete/Discrete Derivative  gainval=1.0  ICPrevScaledInput=0.0  OutMin=[]  OutMax=[]  OutDataType=fixdt(1, 16)  OutScaling=2^-10  DoSatur=off
  Div : Product  Inputs=*/
  Gain : Gain  Gain=-1
  MinMax : MinMax
  Saturation : Saturate  UpperLimit=-1e-6  LowerLimit=-inf
  Terminator : Terminator
  Target_X_TimeToCollision : Outport  VectorParamsAs1DForOutWhenUnconnected=off
  tag scope: AEB_Min_Target_X_Speed=global
  wires:
  Target_X_Distance/1 -> Div/1, Discrete Derivative/1
  Div/1 -> Gain/1
  Gain/1 -> Target_X_TimeToCollision/1
  Discrete Derivative/1 -> Saturation/1
  MinMax/1 -> [AEB_Min_Target_X_Speed]
  Saturation/1 -> MinMax/1, Div/2
  [AEB_Min_Target_X_Speed] -> Terminator/1

== system auto_pilot_udp/AEB/AEB_Logic/Target_XY_TimeToCollision/Target_Y_TimeToCollision_mux ==
  Target_Y_Distance : Inport
  Discrete Derivative1 : simulink/Discrete/Discrete Derivative  gainval=1.0  ICPrevScaledInput=0.0  OutMin=[]  OutMax=[]  OutDataType=fixdt(1, 16)  OutScaling=2^-10  DoSatur=off
  Discrete Derivative2 : simulink/Discrete/Discrete Derivative  gainval=1.0  ICPrevScaledInput=0.0  OutMin=[]  OutMax=[]  OutDataType=fixdt(1, 16)  OutScaling=2^-10  DoSatur=off
  Discrete Derivative3 : simulink/Discrete/Discrete Derivative  gainval=1.0  ICPrevScaledInput=0.0  OutMin=[]  OutMax=[]  OutDataType=fixdt(1, 16)  OutScaling=2^-10  DoSatur=off
  Div1 : Product  Inputs=*/  OutMin=[1e-6]
  Div2 : Product  Inputs=*/
  Gain1 : Gain  Gain=-1
  Gain2 : Gain  Gain=-1
  Lane_Left_Edge_Y_Distance : Constant  Value=1.5
  Lane_Right_Edge_Y_Distance : Constant  Value=-1.5
  MinMax : MinMax
  Saturation : Saturate  UpperLimit=-1e-6  LowerLimit=-inf
  Saturation1 : Saturate  UpperLimit=-1e-6  LowerLimit=-inf
  Sum : Sum  Inputs=+-
  Sum1 : Sum  Inputs=-+
  Terminator : Terminator
  Target_Y_Left_TimeToCollision : Outport  VectorParamsAs1DForOutWhenUnconnected=off
  Target_Y_Right_TimeToCollision : Outport  Port=2  VectorParamsAs1DForOutWhenUnconnected=off
  tag scope: AEB_Min_Target_Y_Speed=global
  wires:
  Discrete Derivative2/1 -> Saturation/1
  Lane_Left_Edge_Y_Distance/1 -> Sum/2
  Target_Y_Distance/1 -> Discrete Derivative3/1, Sum/1, Sum1/2
  Div1/1 -> Gain1/1
  Sum/1 -> Discrete Derivative1/1, Div1/1
  Sum1/1 -> Discrete Derivative2/1, Div2/1
  Discrete Derivative1/1 -> Saturation1/1
  Div2/1 -> Gain2/1
  Gain2/1 -> Target_Y_Left_TimeToCollision/1
  Gain1/1 -> Target_Y_Right_TimeToCollision/1
  Lane_Right_Edge_Y_Distance/1 -> Sum1/1
  Discrete Derivative3/1 -> MinMax/1
  MinMax/1 -> [AEB_Min_Target_Y_Speed]
  Saturation/1 -> Div2/2
  Saturation1/1 -> Div1/2
  [AEB_Min_Target_Y_Speed] -> Terminator/1

== system auto_pilot_udp/OUTPUT/WorldSim_Sensor_Outputs/Subsystem/bsd setection from ostacle recognition ==
  semitrack : Inport
  BSD_matrix_obstalces : Inport  Port=2
  Compare To Constant : simulink/Logic and Bit Operations/Compare To Constant  relop=>  const=30  OutDataTypeStr=boolean
  MATLAB Function3 : MATLAB Function  TreatAsAtomicUnit=on
  Product : Product
  Product1 : Product
  Terminator : Terminator
  Terminator1 : Terminator
  tag scope: BSD_left_ws=global, BSD_right_ws=global
  wires:
  Compare To Constant/1 -> Product1/1, Product/1
  BSD_matrix_obstalces/1 -> MATLAB Function3/1(u)
  Product/1 -> [BSD_left_ws]
  Product1/1 -> [BSD_right_ws]
  MATLAB Function3/2(right) -> Product1/2
  [Vehicle_Speed] -> Compare To Constant/1
  MATLAB Function3/1(left) -> Product/2
  semitrack/1 -> MATLAB Function3/2(semitrack)
  [BSD_left_ws] -> Terminator/1
  [BSD_right_ws] -> Terminator1/1

== system auto_pilot_udp/OUTPUT/WorldSim_Sensor_Outputs/Subsystem/lane marking acquisition ==
  note: . data from ws sensor are y data. sign is negative for right lane, positive for left lane. status = 1 means data are ok. vehicle track is used to make this data as similar as possible to scaner data
  Semitrack : Inport
  Left_lane_marking : Inport  Port=2
  Right_lane_marking : Inport  Port=3
  Bus Creator : BusCreator  Inputs=2
  Constant : Constant  Value=0
  Discrete Filter : DiscreteFilter  Numerator=[butter_b]  Denominator=[butter_a]  SampleTime=1e-3
  Discrete Filter1 : DiscreteFilter  Numerator=[butter_b]  Denominator=[butter_a]  SampleTime=1e-3
  Gain2 : Gain  Gain=-1
  Pulse Generator : DiscretePulseGenerator  PulseType=Time based  Period=1/Sensor_Freq_worldsim  PulseWidth=Sensor_Freq_worldsim*100/1000
  Sum : Sum  Inputs=-+
  Sum1 : Sum  Inputs=-+
  Terminator : Terminator
  Terminator1 : Terminator
  Terminator2 : Terminator
  derivation_speed : Subsystem
  filtering : DiscreteFilter  Numerator=[butter_b]  Denominator=[butter_a]  SampleTime=1e-3
  tag scope: LaneGap_left_ws=global, LaneGap_right_ws=global, LaneGap_speed_left_ws=global, LaneGap_speed_right_ws=global
  wires:
  Semitrack/1 -> Sum/1, Sum1/1
  Gain2/1 -> Sum1/2
  Sum/1 -> derivation_speed/1(Distance), Discrete Filter/1
  Left_lane_marking/1 -> Sum/2
  Sum1/1 -> Discrete Filter1/1
  Discrete Filter/1 -> [LaneGap_left_ws]
  Discrete Filter1/1 -> [LaneGap_right_ws]
  Right_lane_marking/1 -> Gain2/1
  [LaneGap_left_ws] -> Terminator/1
  [LaneGap_right_ws] -> Terminator1/1
  Pulse Generator/1 -> derivation_speed/Trigger
  derivation_speed/1(Speed_of_approaching) -> filtering/1
  filtering/1 -> [LaneGap_speed_left_ws]  "left_lane_approaching_speed"
  Constant/1 -> [LaneGap_speed_right_ws]
  [LaneGap_speed_left_ws] -> Bus Creator/1
  [LaneGap_speed_right_ws] -> Bus Creator/2
  Bus Creator/1 -> Terminator2/1

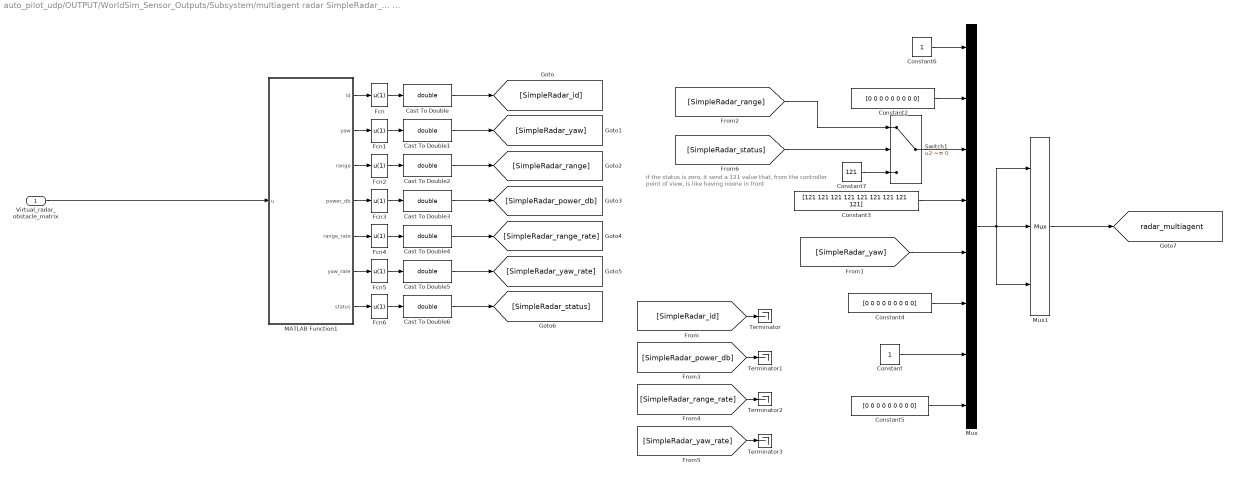
== system auto_pilot_udp/OUTPUT/WorldSim_Sensor_Outputs/Subsystem/multiagent radar SimpleRadar_... are single double representing id, yaw, range, power_db, range_rate, yaw_rate, status ==
  note: if the status is zero, it send a 121 value that,
      | from the controller point of view, is like having noone in front
  Virtual_radar_obstacle_matrix : Inport
  Cast To Double{,1..6} (7 alike) : DataTypeConversion  OutDataTypeStr=double  SaturateOnIntegerOverflow=off  RndMeth=Floor
  Constant : Constant
  Constant2 : Constant  Value=[0 0 0 0 0 0 0 0 0]
  Constant3 : Constant  Value=[121 121 121 121 121 121 121 121 121]
  Constant4 : Constant  Value=[0 0 0 0 0 0 0 0 0]
  Constant5 : Constant  Value=[0 0 0 0 0 0 0 0 0]
  Constant6 : Constant
  Constant7 : Constant  Value=121
  Fcn{,1..6} (7 alike) : Fcn  Expr=u(1)
  MATLAB Function1 : MATLAB Function  TreatAsAtomicUnit=on
  Mux : Mux  Inputs=8
  Mux1 : Mux  Inputs=3
  Switch1 : Switch  Criteria=u2 ~= 0  SaturateOnIntegerOverflow=off  InputSameDT=off
  Terminator{,1..3} (4 alike) : Terminator
  tag scope: radar_multiagent=global
  wires:
  Virtual_radar_obstacle_matrix/1 -> MATLAB Function1/1(u)
  MATLAB Function1/6(yaw_rate) -> Fcn5/1
  Cast To Double3/1 -> [SimpleRadar_power_db]
  Cast To Double5/1 -> [SimpleRadar_yaw_rate]
  MATLAB Function1/1(id) -> Fcn/1
  Fcn4/1 -> Cast To Double4/1
  Cast To Double2/1 -> [SimpleRadar_range]
  Fcn5/1 -> Cast To Double5/1
  MATLAB Function1/2(yaw) -> Fcn1/1
  Cast To Double/1 -> [SimpleRadar_id]
  MATLAB Function1/7(status) -> Fcn6/1
  Fcn1/1 -> Cast To Double1/1
  Fcn6/1 -> Cast To Double6/1
  Fcn/1 -> Cast To Double/1
  Cast To Double4/1 -> [SimpleRadar_range_rate]
  MATLAB Function1/5(range_rate) -> Fcn4/1
  Cast To Double1/1 -> [SimpleRadar_yaw]
  MATLAB Function1/4(power_db) -> Fcn3/1
  Fcn2/1 -> Cast To Double2/1
  Fcn3/1 -> Cast To Double3/1
  MATLAB Function1/3(range) -> Fcn2/1
  Cast To Double6/1 -> [SimpleRadar_status]
  Switch1/1 -> Mux/3
  [SimpleRadar_yaw] -> Mux/5
  [SimpleRadar_status] -> Switch1/2
  Constant3/1 -> Mux/4
  Mux/1 -> Mux1/3, Mux1/1, Mux1/2
  Constant5/1 -> Mux/8
  Constant6/1 -> Mux/1
  Constant/1 -> Mux/7
  Constant4/1 -> Mux/6
  [SimpleRadar_yaw_rate] -> Terminator3/1
  Constant7/1 -> Switch1/3
  Constant2/1 -> Mux/2
  [SimpleRadar_range_rate] -> Terminator2/1
  [SimpleRadar_range] -> Switch1/1
  Mux1/1 -> [radar_multiagent]
  [SimpleRadar_id] -> Terminator/1
  [SimpleRadar_power_db] -> Terminator1/1

== system auto_pilot_udp/OUTPUT/WorldSim_Sensor_Outputs/Subsystem/obstacle detection  ==
  Virtual_camera_obstacle_matrix : Inport
  From1 : From  Commented=on  GotoTag=Obstacles_id
  Gain : Gain  Gain=0.5
  MATLAB Function : MATLAB Function  TreatAsAtomicUnit=on
  MATLAB Function2 : MATLAB Function  TreatAsAtomicUnit=on
  Mux2 : Mux
  Mux3 : Mux  Inputs=3
  Sum : Sum  Inputs=+-
  Terminator{,4..8} (6 alike) : Terminator
  tag scope: Obstacles_nearest_point_x=global, Obstacles_nearest_point_y=global, Obstacles_nearest_point_z=global, Obstacles_type=global, radar_virtual=global
  wires:
  MATLAB Function2/1(tag) -> [Obstacles_type]
  Virtual_camera_obstacle_matrix/1 -> MATLAB Function2/1(u)
  Mux3/1 -> [radar_virtual]
  [Obstacles_nearest_point_x] -> MATLAB Function/1(x)
  [Obstacles_type] -> Mux2/4
  Mux2/1 -> Mux3/2, Mux3/1, Mux3/3
  [Obstacles_nearest_point_y] -> MATLAB Function/2(y)
  MATLAB Function/1(distanceToCollision) -> Mux2/2
  [Obstacles_type] -> Mux2/1
  [Obstacles_nearest_point_z] -> Terminator/1
  MATLAB Function/2(yaw) -> Mux2/3
  MATLAB Function2/3(center_y) -> [Obstacles_nearest_point_y]
  MATLAB Function2/4(center_z) -> [Obstacles_nearest_point_z]
  MATLAB Function2/5(center_rotation_x) -> Terminator6/1
  MATLAB Function2/6(center_rotation_y) -> Terminator7/1
  MATLAB Function2/7(center_rotation_z) -> Terminator8/1
  MATLAB Function2/9(size_y) -> Terminator4/1
  MATLAB Function2/10(size_z) -> Terminator5/1
  MATLAB Function2/8(size_x) -> Gain/1
  MATLAB Function2/2(center_x) -> Sum/1
  Gain/1 -> Sum/2
  Sum/1 -> [Obstacles_nearest_point_x]

== system auto_pilot_udp/OUTPUT/WorldSim_Sensor_Outputs/Subsystem/lane marking acquisition/derivation_speed ==
  Distance : Inport
  Trigger : TriggerPort  VariantControl=Variant  PortDimensions=1
  Discrete Derivative : simulink/Discrete/Discrete Derivative  gainval=1.0  ICPrevScaledInput=0.0  OutMin=[]  OutMax=[]  OutDataType=fixdt(1, 16)  OutScaling=2^-10  DoSatur=off
  Gain : Gain  Gain=-1
  Speed_of_approaching : Outport
  wires:
  Discrete Derivative/1 -> Gain/1
  Gain/1 -> Speed_of_approaching/1
  Distance/1 -> Discrete Derivative/1

== matlab function auto_pilot_udp/OUTPUT/WorldSim_Sensor_Outputs/Subsystem/multiagent radar SimpleRadar_... are single double representing id, yaw, range, power_db, range_rate, yaw_rate, status/MATLAB Function1 ==
  data: u input; id output; yaw output; range output; power_db output; range_rate output; yaw_rate output; status output
function [id, yaw, range, power_db, range_rate, yaw_rate,status] = fcn(u)

id = u(:,1);
yaw = u(:,2);
range = u(:,3);
power_db = u(:,4);
range_rate = u(:,5);
yaw_rate = u(:,6);
status = u(:,7);

== matlab function auto_pilot_udp/OUTPUT/WorldSim_Sensor_Outputs/Subsystem/obstacle detection /MATLAB Function2 ==
  data: u input; tag output; center_x output; center_y output; center_z output; center_rotation_x output; center_rotation_y output; center_rotation_z output; size_x output; size_y output; size_z output
function [tag, center_x, center_y, center_z, center_rotation_x, center_rotation_y, center_rotation_z, size_x, size_y, size_z] = fcn(u)

% this is the id tag that is assigned by ws at every scenario load
tag = (u(1,:))';
center_x = (u(2,:))';
center_y = (u(3,:))';
center_z = (u(4,:))';
center_rotation_x = (u(5,:))';
center_rotation_y = (u(6,:))';
center_rotation_z = (u(7,:))';
size_x = (u(8,:))';
size_y = (u(9,:))';
size_z = (u(10,:))';

%% identification of nearest box

% [index,index2]=min(u(:,3));
% 
% id = u(index,1);
% type = u(index,2);
% center_x = u(index,3);
% center_y = u(index,4);
% center_z = u(index,5);
% width = u(index,6);
% height = u(index,7);

== matlab function auto_pilot_udp/OUTPUT/WorldSim_Sensor_Outputs/Subsystem/obstacle detection /MATLAB Function ==
  data: x input; distanceToCollision output; y input; yaw output
function [distanceToCollision, yaw] = fcn(x, y)

x(x==0)=121;
y(y==0)=121;

yaw = atan(y./x);
distanceToCollision=x./cos(yaw);
distanceToCollision(x==121)=121;

== matlab function auto_pilot_udp/AEB/AEB_Inputs/MATLAB Function ==
  data: u input; y output
function y = fcn(u)

y = u;
y(u==121)=0;

== matlab function auto_pilot_udp/AEB/AEB_Inputs/MATLAB Function1 ==
  data: u input; y output
function y = fcn(u)

y = u;
y(u==121)=0;

== matlab function auto_pilot_udp/OUTPUT/WorldSim_Sensor_Outputs/Subsystem/bsd setection from ostacle recognition/MATLAB Function3 ==
  data: u input; semitrack input; left output; right output
function [left, right] = fcn(u, semitrack)
left=0;
right=0;

% [x,index] = min(nonzeros(u(:,3)));
x = (u(2,:))';
y = (u(3,:))';
% yaw = atan(y./x);
% distanceToCollision=x./cos(yaw);
index_left=find((y < -semitrack).*(y > -5),1);
index_right=find((y > semitrack).*(y < 5),1);
% .*(y > -3).*(x < 25)
if (~isempty(index_left))
    left = 1;
end
if (~isempty(index_right))
    right=1;
end

== matlab function auto_pilot_udp/OUTPUT/WorldSim_Sensor_Outputs/manipulation_of_objects1 ==
  data: complete_obstacles_matrix input; filtered_matrix output; detected_objects input
function filtered_matrix = fcn(complete_obstacles_matrix, detected_objects)

% computations

filtered_matrix = complete_obstacles_matrix;

filtered_matrix(:,((detected_objects+1):size(filtered_matrix,2))) = 0;

== matlab function auto_pilot_udp/AP/AP_Logic/MATLAB Function ==
  data: u input; y output
function y = fcn(u)

if u == 0
    y=1e-6;
else
    y=u;
end

end

== matlab function auto_pilot_udp/ACC/ACC_Logic/ACC_Target_Acquisition/SensorTargets_300000_InCurvedLane_mux/MATLAB Function ==
  data: Front_Axle_Steer input; Radius output; Rn output; wheelbase input; SensorTargets_300000_LongitudinalDistance input; SensorTargets_300000_LateralDistance input
function [Radius,Rn]= fcn(Front_Axle_Steer,wheelbase,SensorTargets_300000_LongitudinalDistance,SensorTargets_300000_LateralDistance)
%% Calc corner radius from steer at front axle
Radius = wheelbase./sin(Front_Axle_Steer) ; % (m)

%% Calc center of cirle coordinates (orgin reference at center of front axle)
yc = wheelbase./tan(Front_Axle_Steer) ; %(rad)
xc = -wheelbase ; %(m)

%% Calc target distance from circle center 
yn = SensorTargets_300000_LateralDistance ; %(m)
xn = SensorTargets_300000_LongitudinalDistance ; %(m)

Rn = sqrt((yn-yc).^2+(xn-xc).^2) ; %(m)

== matlab function auto_pilot_udp/OUTPUT/WorldSim_Sensor_Outputs/MATLAB Function ==
  data: lane_coefficiants input; left_lane_distance output; right_lane_distance output
function [left_lane_distance, right_lane_distance] = fcn(lane_coefficiants)

left_lane_distance = lane_coefficiants(1,1);
right_lane_distance = lane_coefficiants(2,1);
